simulink model "Simulinkproyecto"  (R2019b)
settings: Solver=VariableStepAuto  StartTime=0.0  StopTime=100  RelTol=1e-3
values from neighbouring files (symbols this model uses):
  S = (1-z^-1)*(1+s1*z^-1)    [Controlador.m]
libraries: cstblocks x10
settings Model: Creator=Admin  LastModifiedBy=Admin

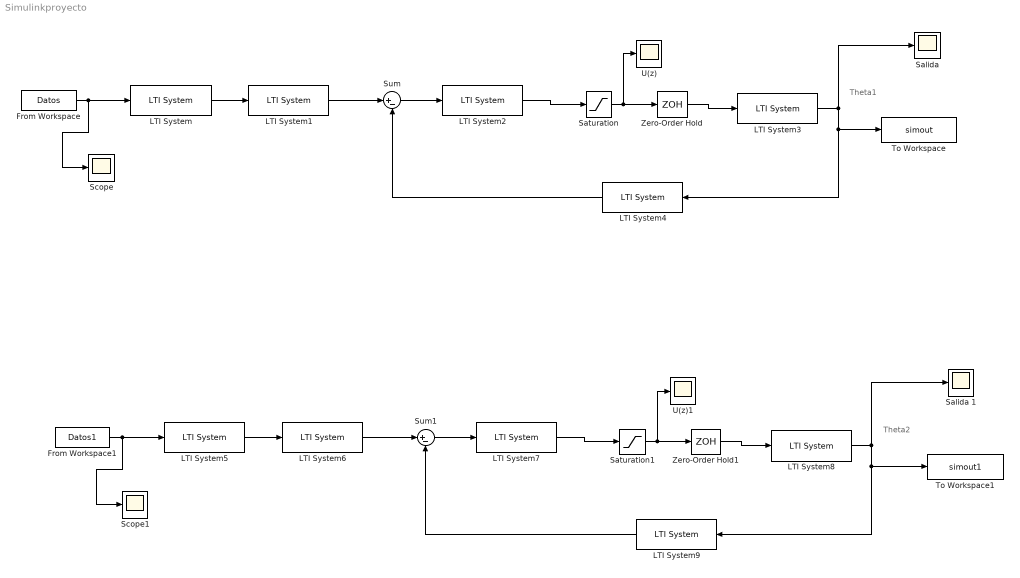
== system Simulinkproyecto ==
  note: Theta1
  note: Theta2
  From Workspace : FromWorkspace  VariableName=Datos  SampleTime=0
  From Workspace1 : FromWorkspace  VariableName=Datos1  SampleTime=0
  LTI System : cstblocks/LTI System  sys=prez  IC=[]
  LTI System{1,4,6,9} (4 alike) : cstblocks/LTI System  sys=R  IC=[]
  LTI System2 : cstblocks/LTI System  sys=1/S  IC=[]
  LTI System3 : cstblocks/LTI System  sys=G  IC=[]
  LTI System5 : cstblocks/LTI System  sys=prez  IC=[]
  LTI System7 : cstblocks/LTI System  sys=1/S  IC=[]
  LTI System8 : cstblocks/LTI System  sys=G  IC=[]
  "Salida " : Scope
  Salida 1 : Scope
  Saturation : Saturate  UpperLimit=12  LowerLimit=0
  Saturation1 : Saturate  UpperLimit=12  LowerLimit=0
  Scope : Scope
  Scope1 : Scope
  Sum : Sum  Inputs=|+-
  Sum1 : Sum  Inputs=|+-
  To Workspace : ToWorkspace  VariableName=simout  SaveFormat=Structure With Time  SampleTime=-1
  To Workspace1 : ToWorkspace  VariableName=simout1  SaveFormat=Structure With Time  SampleTime=-1
  U(z) : Scope
  U(z)1 : Scope
  Zero-Order Hold : ZeroOrderHold  SampleTime=0.001
  Zero-Order Hold1 : ZeroOrderHold  SampleTime=0.001
  wires:
  From Workspace/1 -> Scope/1, LTI System/1
  LTI System/1 -> LTI System1/1
  LTI System1/1 -> Sum/1
  Sum/1 -> LTI System2/1
  LTI System2/1 -> Saturation/1
  Saturation/1 -> U(z)/1, Zero-Order Hold/1
  Zero-Order Hold/1 -> LTI System3/1
  LTI System3/1 -> "Salida "/1, To Workspace/1, LTI System4/1
  LTI System4/1 -> Sum/2
  From Workspace1/1 -> Scope1/1, LTI System5/1
  LTI System7/1 -> Saturation1/1
  Zero-Order Hold1/1 -> LTI System8/1
  Sum1/1 -> LTI System7/1
  LTI System9/1 -> Sum1/2
  LTI System6/1 -> Sum1/1
  Saturation1/1 -> U(z)1/1, Zero-Order Hold1/1
  LTI System8/1 -> To Workspace1/1, LTI System9/1, Salida 1/1
  LTI System5/1 -> LTI System6/1
